simulink model "RLS"  (R2022a)
settings: Solver=FixedStepAuto  StartTime=0.0  StopTime=3  FixedStep=0.0003  MaxStep=0.0003  RelTol=1e-12  AbsTol=1e-9
values from neighbouring files (symbols this model uses):
  L = dims(2)    [LMS_IIRcompute.m]    (also in d_phi.m = args.beam.L; phi.m = args.beam.L)
  M = dims(1)    [LMS_IIRcompute.m]    (also in computeMCK.m = zeros(args.n); magPhase.m = zeros(1,length(freq_range)))
undefined symbols (not defined in the file or in its folder): den_lpf, filter_coefficients, model, num_lpf
libraries: matrix_library x3, simulink x2
settings Model: Creator=jdkoc  LastModifiedBy=jdkoc
settings DebuggingCC: InheritedTsInSrcMsg=none

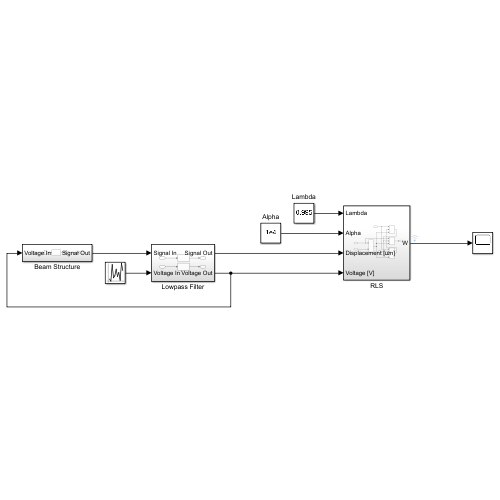
[thumbnail: Simulink's stored preview of the top-level diagram]
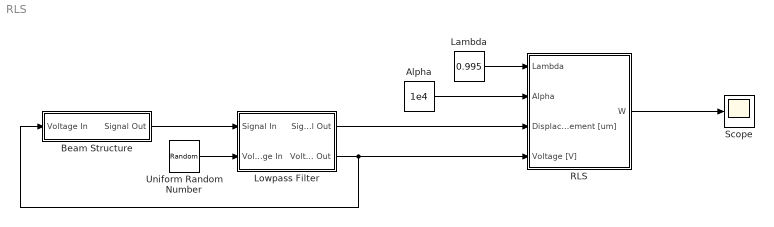
== system RLS ==
  Alpha : Constant  Value=1e4
  Beam Structure : Subsystem
  Lambda : Constant  Value=0.995
  Lowpass Filter : Subsystem
  RLS : Subsystem
  Scope : Scope
  Uniform Random Number : UniformRandomNumber
  wires:
  Lambda/1 -> RLS/1(Lambda)
  Alpha/1 -> RLS/2(Alpha)
  RLS/1(W) -> Scope/1
  Lowpass Filter/1(Signal Out) -> RLS/3(Displacement [um])
  Beam Structure/1(Signal Out) -> Lowpass Filter/1(Signal In)
  Lowpass Filter/2(Voltage Out) -> RLS/4(Voltage [V]), Beam Structure/1(Voltage In)
  Uniform Random Number/1 -> Lowpass Filter/2(Voltage In)

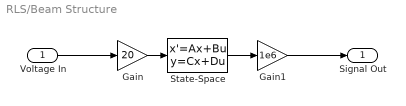
== system RLS/Beam Structure ==
  Voltage In : Inport
  Gain : Gain  Gain=20
  Gain1 : Gain  Gain=1e6
  State-Space : StateSpace  A=model.dynamics.ss.A  B=model.dynamics.ss.B*[1;0]  C=model.dynamics.ss.C  D=model.dynamics.ss.D*[1;0]  InitialCondition=0
  Signal Out : Outport
  wires:
  Voltage In/1 -> Gain/1
  Gain1/1 -> Signal Out/1
  Gain/1 -> State-Space/1
  State-Space/1 -> Gain1/1

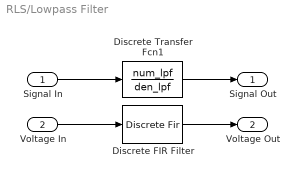
== system RLS/Lowpass Filter ==
  Signal In : Inport
  Voltage In : Inport  Port=2
  Discrete Transfer Fcn1 : DiscreteTransferFcn  Numerator=num_lpf  Denominator=den_lpf
  Discrete FIR Filter : DiscreteFir  Coefficients=filter_coefficients
  Signal Out : Outport
  Voltage Out : Outport  Port=2
  wires:
  Signal In/1 -> Discrete Transfer Fcn1/1
  Discrete Transfer Fcn1/1 -> Signal Out/1
  Discrete FIR Filter/1 -> Voltage Out/1
  Voltage In/1 -> Discrete FIR Filter/1

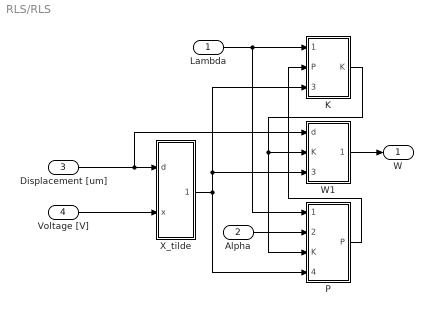
== system RLS/RLS ==
  Lambda : Inport
  Alpha : Inport  Port=2
  Displacement [um] : Inport  Port=3
  Voltage [V] : Inport  Port=4
  K : Subsystem
  P : Subsystem
  W1 : Subsystem
  X_tilde : Subsystem
  W : Outport
  wires:
  K/1(K) -> P/3(K), W1/2(K)
  P/1(P) -> K/2(P)
  X_tilde/1(X_tilde) -> K/3(X_tilde), W1/3(X_tilde), P/4(X_tilde)
  Lambda/1 -> P/1(Lambda), K/1(Lambda)
  W1/1(W1) -> W/1
  Alpha/1 -> P/2(Alpha)
  Displacement [um]/1 -> W1/1(d), X_tilde/1(d)
  Voltage [V]/1 -> X_tilde/2(x)

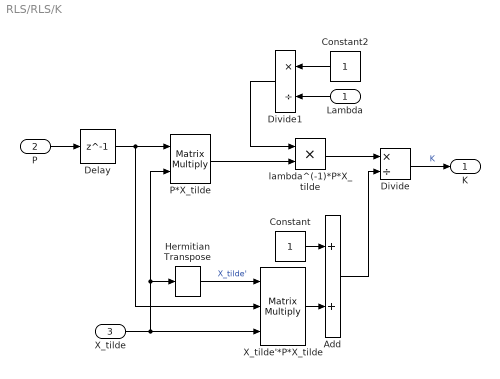
== system RLS/RLS/K ==
  Lambda : Inport
  P : Inport  Port=2
  X_tilde : Inport  Port=3
  Add : Sum
  Constant : Constant
  Constant2 : Constant
  Delay : Delay  DelayLength=1
  Divide : Product  Inputs=*/
  Divide1 : Product  Inputs=*/
  Hermitian Transpose : matrix_library/Hermitian Transpose
      settings: SourceProductBaseCode=SL
  P*X_tilde : Product  Multiplication=Matrix(*)
  X_tilde'*P*X_tilde : Product  Inputs=3  Multiplication=Matrix(*)
  lambda^(-1)*P*X_tilde : Product
  K : Outport
  wires:
  Constant2/1 -> Divide1/1
  Divide1/1 -> lambda^(-1)*P*X_tilde/1
  X_tilde/1 -> P*X_tilde/2, Hermitian Transpose/1, X_tilde'*P*X_tilde/3
  Divide/1 -> K/1  "K"
  Lambda/1 -> Divide1/2
  X_tilde'*P*X_tilde/1 -> Add/2
  Constant/1 -> Add/1
  Add/1 -> Divide/2
  P*X_tilde/1 -> lambda^(-1)*P*X_tilde/2
  lambda^(-1)*P*X_tilde/1 -> Divide/1
  Hermitian Transpose/1 -> X_tilde'*P*X_tilde/1  "X_tilde'"
  P/1 -> Delay/1
  Delay/1 -> X_tilde'*P*X_tilde/2, P*X_tilde/1

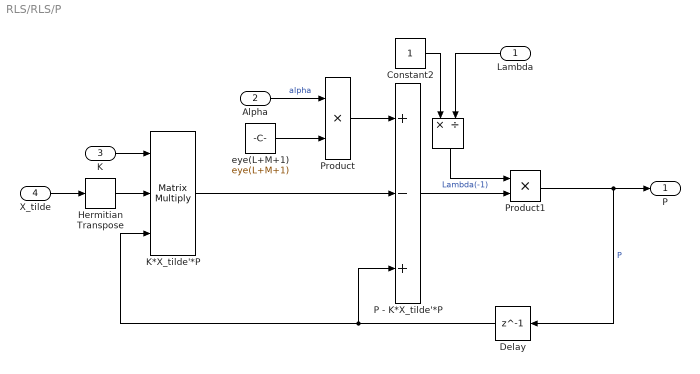
== system RLS/RLS/P ==
  Lambda : Inport  PortDimensions=1
  Alpha : Inport  Port=2  PortDimensions=1
  K : Inport  Port=3  PortDimensions=[L+M+1,1]
  X_tilde : Inport  Port=4  PortDimensions=[L+M+1,1]
  " " : Product  Inputs=*/
  Constant2 : Constant
  Delay : Delay  DelayLength=1
  Hermitian Transpose : matrix_library/Hermitian Transpose
      settings: SourceProductBaseCode=SL
  K*X_tilde'*P : Product  Inputs=3  Multiplication=Matrix(*)  InputSameDT=on
  P - K*X_tilde'*P : Sum  Inputs=+-+
  Product : Product
  Product1 : Product
  eye(L+M+1) : Constant  Value=eye(L+M+1)
  P : Outport
  wires:
  Hermitian Transpose/1 -> K*X_tilde'*P/2
  P - K*X_tilde'*P/1 -> Product1/2
  X_tilde/1 -> Hermitian Transpose/1
  Constant2/1 -> " "/1
  " "/1 -> Product1/1  "Lambda(-1)"
  eye(L+M+1)/1 -> Product/2
  K*X_tilde'*P/1 -> P - K*X_tilde'*P/2
  K/1 -> K*X_tilde'*P/1
  Product1/1 -> P/1, Delay/1  "P"
  Alpha/1 -> Product/1  "alpha"
  Lambda/1 -> " "/2
  Product/1 -> P - K*X_tilde'*P/1
  Delay/1 -> P - K*X_tilde'*P/3, K*X_tilde'*P/3

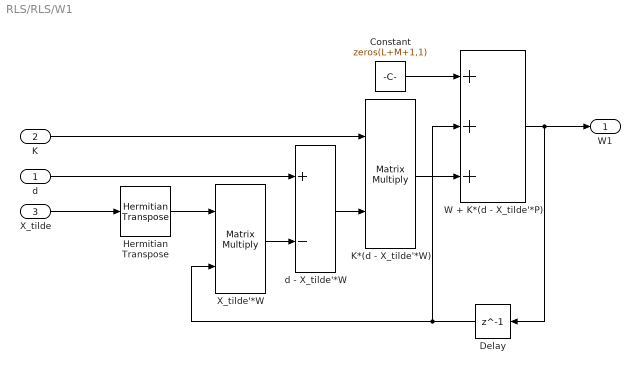
== system RLS/RLS/W1 ==
  d : Inport
  K : Inport  Port=2
  X_tilde : Inport  Port=3
  Constant : Constant  Value=zeros(L+M+1,1)
  Delay : Delay  DelayLength=1
  Hermitian Transpose : matrix_library/Hermitian Transpose
      settings: SourceProductBaseCode=SL
  K*(d - X_tilde'*W) : Product  Multiplication=Matrix(*)
  W + K*(d - X_tilde'*P) : Sum  Inputs=+++
  X_tilde'*W : Product  Multiplication=Matrix(*)
  d - X_tilde'*W : Sum  Inputs=+-
  W1 : Outport
  wires:
  d - X_tilde'*W/1 -> K*(d - X_tilde'*W)/2
  K/1 -> K*(d - X_tilde'*W)/1
  X_tilde'*W/1 -> d - X_tilde'*W/2
  K*(d - X_tilde'*W)/1 -> W + K*(d - X_tilde'*P)/3
  W + K*(d - X_tilde'*P)/1 -> Delay/1, W1/1
  X_tilde/1 -> Hermitian Transpose/1
  Hermitian Transpose/1 -> X_tilde'*W/1
  d/1 -> d - X_tilde'*W/1
  Constant/1 -> W + K*(d - X_tilde'*P)/1
  Delay/1 -> W + K*(d - X_tilde'*P)/2, X_tilde'*W/2

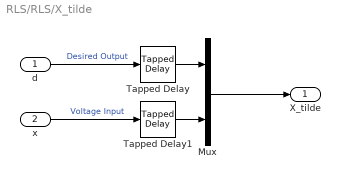
== system RLS/RLS/X_tilde ==
  d : Inport
  x : Inport  Port=2
  Mux : Mux  Inputs=2
  Tapped Delay : simulink/Discrete/Tapped Delay  vinit=0.0  samptime=-1  NumDelays=L  DelayOrder=Newest  includeCurrent=off
  Tapped Delay1 : simulink/Discrete/Tapped Delay  vinit=0.0  samptime=-1  NumDelays=M  DelayOrder=Newest  includeCurrent=on
  X_tilde : Outport
  wires:
  d/1 -> Tapped Delay/1  "Desired Output"
  x/1 -> Tapped Delay1/1  "Voltage Input"
  Mux/1 -> X_tilde/1
  Tapped Delay1/1 -> Mux/2
  Tapped Delay/1 -> Mux/1
